simulink model "LQR_non_linear"  (R2017b)
settings: Solver=VariableStepAuto  StartTime=0.0  StopTime=100  RelTol=1e-3
values from neighbouring files (symbols this model uses):
  g = 9.8    [Controls_project.m]
  K = lqr(A,B,q,r)    [Controls_project.m]
  l1 = 20    [Controls_project.m]
  l2 = 10    [Controls_project.m]
  M = 1000    [Controls_project.m]
  m1 = 100    [Controls_project.m]
  m2 = 100    [Controls_project.m]
settings Model: Creator=Adheesh  LastModifiedBy=Adheesh

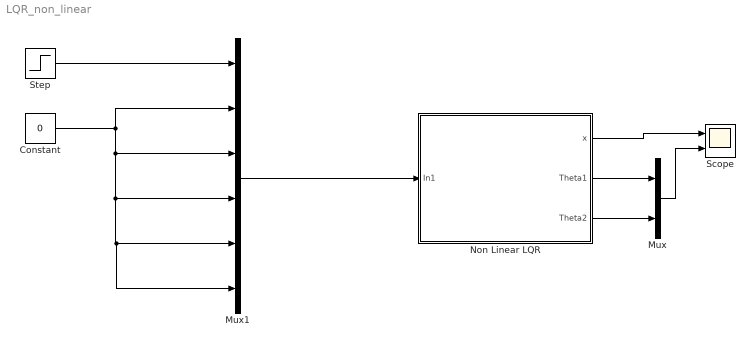
== system LQR_non_linear ==
  Constant : Constant  Value=0
  Mux : Mux  Inputs=2
  Mux1 : Mux  Inputs=6
  Non Linear LQR : Subsystem
  Scope : Scope  NumInputPorts=2
  Step : Step  SampleTime=0
  wires:
  Non Linear LQR/1("x ") -> Scope/1
  Non Linear LQR/2(Theta1) -> Mux/1
  Non Linear LQR/3(Theta2) -> Mux/2
  Mux/1 -> Scope/2
  Constant/1 -> Mux1/6, Mux1/5, Mux1/4, Mux1/3, Mux1/2
  Step/1 -> Mux1/1
  Mux1/1 -> Non Linear LQR/1(In1)

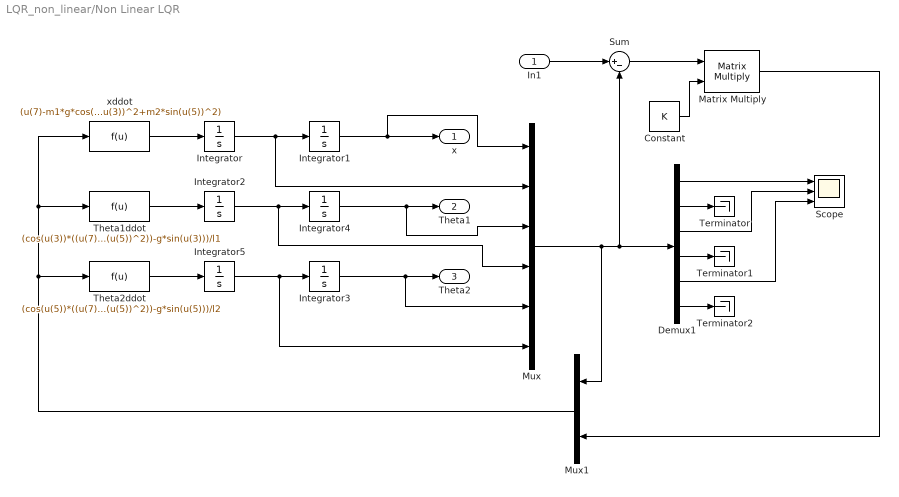
== system LQR_non_linear/Non Linear LQR ==
  In1 : Inport
  Constant : Constant  Value=K
  Demux1 : Demux  Outputs=6
  Integrator{,1..5} (6 alike) : Integrator
  Matrix Multiply : Product  Multiplication=Matrix(*)
  Mux : Mux  Inputs=6
  Mux1 : Mux  Inputs=2
  Scope : Scope  NumInputPorts=3
  Sum : Sum  Inputs=|+-
  Terminator : Terminator
  Terminator1 : Terminator
  Terminator2 : Terminator
  Theta1ddot : Fcn  Expr=(cos(u(3))*((u(7)-m1*g*cos(u(3))*sin(u(3))-m2*g*cos(u(5))*sin(u(5))-m1*l1*sin(u(3))*u(4)^2-m2*l2*sin(u(5))*u(6)^2)/(M+m1*sin(u(3))^2+m2*sin(u(5))^2))-g*sin(u(3)))/l1
  "Theta2ddot " : Fcn  Expr=(cos(u(5))*((u(7)-m1*g*cos(u(3))*sin(u(3))-m2*g*cos(u(5))*sin(u(5))-m1*l1*sin(u(3))*u(4)^2-m2*l2*sin(u(5))*u(6)^2)/(M+m1*sin(u(3))^2+m2*sin(u(5))^2))-g*sin(u(5)))/l2
  "xddot " : Fcn  Expr=(u(7)-m1*g*cos(u(3))*sin(u(3))-m2*g*cos(u(5))*sin(u(5))-m1*l1*sin(u(3))*u(4)^2-m2*l2*sin(u(5))*u(6)^2)/(M+m1*sin(u(3))^2+m2*sin(u(5))^2)
  "x " : Outport
  Theta1 : Outport  Port=2
  Theta2 : Outport  Port=3
  wires:
  Constant/1 -> Matrix Multiply/2
  Demux1/2 -> Terminator/1
  Sum/1 -> Matrix Multiply/1
  Demux1/5 -> Scope/3
  Integrator5/1 -> Mux/6, Integrator3/1
  Demux1/4 -> Terminator1/1
  Demux1/6 -> Terminator2/1
  Demux1/1 -> Scope/1
  In1/1 -> Sum/1
  Matrix Multiply/1 -> Mux1/2
  "Theta2ddot "/1 -> Integrator5/1
  Integrator2/1 -> Mux/4, Integrator4/1
  Integrator4/1 -> Theta1/1, Mux/3
  Mux1/1 -> "Theta2ddot "/1, Theta1ddot/1, "xddot "/1
  Mux/1 -> Sum/2, Demux1/1, Mux1/1
  Demux1/3 -> Scope/2
  Integrator/1 -> Mux/2, Integrator1/1
  "xddot "/1 -> Integrator/1
  Integrator1/1 -> Mux/1, "x "/1
  Theta1ddot/1 -> Integrator2/1
  Integrator3/1 -> Theta2/1, Mux/5
